simulink model "Mutant_19_of_purePursuitUSCityCopia"  (R2020a)
settings: Solver=FixedStepAuto  StartTime=0.0  StopTime=Ts  FixedStep=0.001  RelTol=1e-3
PreLoadFcn:
  | setUpPurePursuitUSCity
model workspace (MAT data in the model file):
  firstWarning = 0
  originalScenarioChecksum = 'F73A6DA3C723D3CA73A6F931B7A52A9C'
undefined symbols (not defined in the file): angVelGain, approximationReductionGain, L, ld, magnitude, minimalSpeed, nominalSpeed, psi_1, psi_2, psi_o, slope_x1, slope_x2, slope_y1, slope_y2, x_1, x_2, X_o, xRef, y_1, y_2, Y_o, yRef
libraries: simulink x15, autolibutils x4, autolibshared x3, robotalgslib x1
(part 3 of 3)

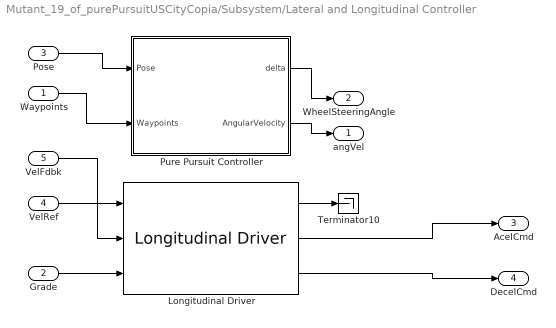
== system Mutant_19_of_purePursuitUSCityCopia/Subsystem/Lateral and Longitudinal Controller ==
  Waypoints : Inport
  Grade : Inport  Port=2
  Pose : Inport  Port=3
  VelRef : Inport  Port=4
  VelFdbk : Inport  Port=5
  Longitudinal Driver : autolibshared/Longitudinal Driver  extAccelOvr=off  extDecelOvr=off  extAccelHld=off  extDecelHld=off  extAccelZero=off  extDecelZero=off  cntrlType=PI  shftType=None  velUnits=m/s  gearOut=off  Kp=700  Ki=1  Kff=.1  Kg=0  VehVelVec=[0 100]  KffVec=[.1 .1]  KpVec=[10 10]  KiVec=[5 5]  KgVec=[0 0]  m=1500  Kpt=3000  tau=.1  L=2  aR=200  bR=2.5  cR=.5  g=9.81  vnom=9  Kaw=1  tauerr=.01  tauPt=2  GearInit=0  tShift=.1  pdlVec=[0.1 0.4 0.5 0.9]  upShftTbl=[-1 12.9375 26.4375 39.9375 51.18749999999999 62.4375 72.84375 83.25;-1 16.3125 29.8125 43.3125 54.5624 65.8125 76.78125 87.75;-1 19.6875 33.1875 46.68749999999999 57.9375 69.1875 80.71875 92.25;-1 33 52.5 77.25 100.5 138.75 161.875 185]  dwnShftTbl=[1 9.5625 23.0625 36.5625 47.8125 59.0625 68.90625 78.75;1 12.9375 26.4375 39.9375 51.18749999999999 62.4375 72.84375 83.25;1 16.3125 29.8125 43.3125 54.562499 65.8125 76.78125 87.75;1 19.6875 33.1875 46.68749999999999 57.9375 69.1875 80.71875 92.25]  tClutch=.5  tRev=.5  tPark=120  aMode=2  UpGearVec="[0  1  2  3  4  5  6  7]"  DownGearVec="[1  2  3  4  5  6  7  8]"
      settings: SourceProductBaseCode=PW,MT,VE,VP
  Pure Pursuit Controller : Subsystem
  Terminator10 : Terminator
  angVel : Outport
  WheelSteeringAngle : Outport  Port=2
  AcelCmd : Outport  Port=3
  DecelCmd : Outport  Port=4
  wires:
  Pure Pursuit Controller/1(delta) -> WheelSteeringAngle/1
  Waypoints/1 -> Pure Pursuit Controller/2(Waypoints)
  Pose/1 -> Pure Pursuit Controller/1(Pose)
  Grade/1 -> Longitudinal Driver/3
  VelRef/1 -> Longitudinal Driver/1
  VelFdbk/1 -> Longitudinal Driver/2
  Longitudinal Driver/1 -> Terminator10/1
  Pure Pursuit Controller/2(AngularVelocity) -> angVel/1
  Longitudinal Driver/2 -> AcelCmd/1
  Longitudinal Driver/3 -> DecelCmd/1

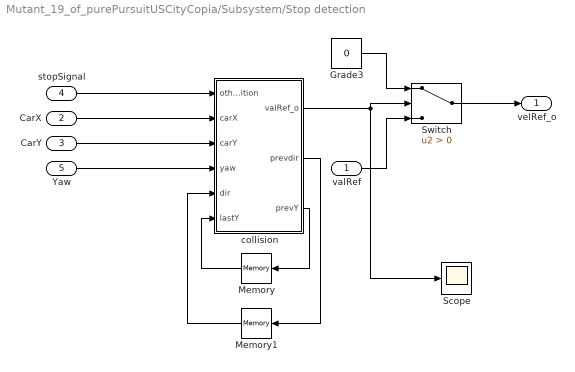
== system Mutant_19_of_purePursuitUSCityCopia/Subsystem/Stop detection ==
  valRef : Inport
  CarX : Inport  Port=2
  CarY : Inport  Port=3
  stopSignal : Inport  Port=4
  Yaw : Inport  Port=5
  Grade3 : Constant  Value=0
  Memory : Memory
  Memory1 : Memory
  Scope : Scope
  Switch : Switch  Criteria=u2 > Threshold
  collision : MATLAB Function  TreatAsAtomicUnit=on
  velRef_o : Outport
  wires:
  Switch/1 -> velRef_o/1
  valRef/1 -> Switch/3
  Grade3/1 -> Switch/1
  collision/1(valRef_o) -> Switch/2, Scope/1
  stopSignal/1 -> collision/1(otherCarPosition)
  CarX/1 -> collision/2(carX)
  CarY/1 -> collision/3(carY)
  Yaw/1 -> collision/4(yaw)
  collision/2(prevdir) -> Memory1/1
  collision/3(prevY) -> Memory/1
  Memory/1 -> collision/6(lastY)
  Memory1/1 -> collision/5(dir)

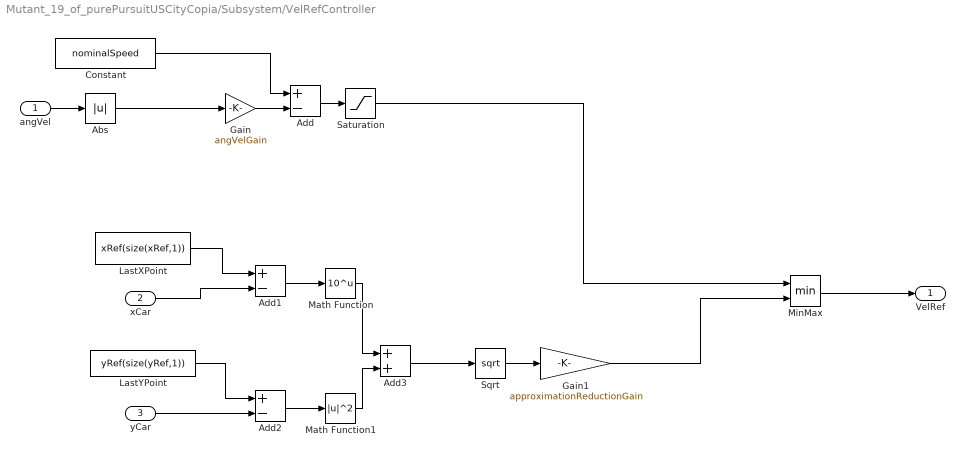
== system Mutant_19_of_purePursuitUSCityCopia/Subsystem/VelRefController ==
  angVel : Inport
  xCar : Inport  Port=2
  yCar : Inport  Port=3
  Abs : Abs
  Add : Sum  Inputs=+-
  Add1 : Sum  Inputs=+-
  Add2 : Sum  Inputs=+-
  Add3 : Sum
  Constant : Constant  Value=nominalSpeed
  Gain : Gain  Gain=angVelGain
  Gain1 : Gain  Gain=approximationReductionGain
  LastXPoint : Constant  Value=xRef(size(xRef,1))  SampleTime=0.1
  LastYPoint : Constant  Value=yRef(size(yRef,1))  SampleTime=0.1
  Math Function : Math  Operator=10^u  SaturateOnIntegerOverflow=on
  Math Function1 : Math  Operator=magnitude^2  SaturateOnIntegerOverflow=on
  MinMax : MinMax  Inputs=2
  Saturation : Saturate  UpperLimit=15  LowerLimit=minimalSpeed
  Sqrt : Sqrt  SaturateOnIntegerOverflow=on
  VelRef : Outport
  wires:
  angVel/1 -> Abs/1
  Gain/1 -> Add/2
  Abs/1 -> Gain/1
  Constant/1 -> Add/1
  Add/1 -> Saturation/1
  LastYPoint/1 -> Add2/1
  Math Function1/1 -> Add3/2
  Add3/1 -> Sqrt/1
  LastXPoint/1 -> Add1/1
  Math Function/1 -> Add3/1
  Add2/1 -> Math Function1/1
  yCar/1 -> Add2/2
  Add1/1 -> Math Function/1
  Sqrt/1 -> Gain1/1
  xCar/1 -> Add1/2
  Gain1/1 -> MinMax/2
  Saturation/1 -> MinMax/1
  MinMax/1 -> VelRef/1

== system Mutant_19_of_purePursuitUSCityCopia/Powertrain & Driveline/Driveline/AWD ==
  TPowertrain : Inport
  AWD : Gain  Gain=[1;1;1;1]./2
  TAxles : Outport  VectorParamsAs1DForOutWhenUnconnected=off
  wires:
  TPowertrain/1 -> AWD/1
  AWD/1 -> TAxles/1

== system Mutant_19_of_purePursuitUSCityCopia/Powertrain & Driveline/Driveline/FWD ==
  TPowertrain : Inport
  FWD : Gain  Gain=[1;1;0;0]
  TAxles : Outport  VectorParamsAs1DForOutWhenUnconnected=off
  wires:
  FWD/1 -> TAxles/1
  TPowertrain/1 -> FWD/1

== system Mutant_19_of_purePursuitUSCityCopia/Powertrain & Driveline/Driveline/RWD ==
  TPowertrain : Inport
  RWD : Gain  Gain=[0;0;1;1]
  TAxles : Outport  VectorParamsAs1DForOutWhenUnconnected=off
  wires:
  TPowertrain/1 -> RWD/1
  RWD/1 -> TAxles/1

== system Mutant_19_of_purePursuitUSCityCopia/Subsystem/Lateral and Longitudinal Controller/Pure Pursuit Controller ==
  note: The subsystem implements a Pure Pursuit controller. The "Pure Pursuit" block calculates the target direction and the "Wheel Steering Angle Formulation" block calculates the wheel steering angle.
  Pose : Inport
  Waypoints : Inport  Port=2
  Pure Pursuit : robotalgslib/Pure Pursuit  DesiredLinearVelocity=0.5  MaxAngularVelocity=1.0  LookaheadDistance=ld  TargetDirPort=on  SimulateUsing=Code generation
  Terminator6 : Terminator
  Terminator7 : Terminator
  Wheel Steering Angle Formulation : Subsystem  mask{L=L, ld=ld}
      mask prompts: L "Bicycle length"; ld "Lookahead distance"
      mask TypeOptions L: Bicycle length/Value
      mask TypeOptions ld: Lookahead distance/Value
      mask Display:
      | image("GeometryMask.png")
      | port_label('input', 1, 'alpha')
      | port_label('output', 1, 'delta')
  delta : Outport
  AngularVelocity : Outport  Port=2
  wires:
  Wheel Steering Angle Formulation/1(Al) -> delta/1
  Pure Pursuit/3 -> Wheel Steering Angle Formulation/1(alpha)
  Waypoints/1 -> Pure Pursuit/2
  Pure Pursuit/2 -> AngularVelocity/1, Terminator7/1
  Pose/1 -> Pure Pursuit/1
  Pure Pursuit/1 -> Terminator6/1

== system Mutant_19_of_purePursuitUSCityCopia/Subsystem/Lateral and Longitudinal Controller/Pure Pursuit Controller/Wheel Steering Angle Formulation ==
  alpha : Inport
  Bicycle length : Constant  Value=L
  Constant : Constant  Value=2
  Divide : Product  Inputs=*/
  Lookahead distance : Constant  Value=ld
  Product : Product
  Product1 : Product
  Sine Wave : Sin  TimeSource=Use external signal  SampleTime=0
  Trigonometric Function : Trigonometry  Operator=atan
  Al : Outport
  wires:
  Sine Wave/1 -> Product1/2
  Bicycle length/1 -> Product/2
  Constant/1 -> Product/1
  Product1/1 -> Divide/1
  Product/1 -> Product1/1
  Divide/1 -> Trigonometric Function/1
  Trigonometric Function/1 -> Al/1
  alpha/1 -> Sine Wave/1
  Lookahead distance/1 -> Divide/2

== matlab function Mutant_19_of_purePursuitUSCityCopia/Subsystem/Stop detection/collision ==
  data: valRef_o output; otherCarPosition input; carX input; carY input; yaw input; prevdir output; prevY output; dir input; lastY input
function [valRef_o,prevdir,prevY] = fcn(otherCarPosition,carX,carY ,yaw, dir, lastY)
%     ret=0;
%     for i=1:(size(waypoints,2)/2)
%         if waypoints(1,2*i-1)-data(1,1)<10 && waypoints(1,2*i)-data(1,2)<10 && waypoints(1,2*i-1)-data(1,1)>-10 && waypoints(1,2*i)-data(1,2)>-10 
%             ret=1;
%         end
%     end
    detectedCar=0;
    i=1;
    distanceX=0;
    distanceY=0;
    while i<=(size(otherCarPosition,2)/2) && detectedCar==0
        distanceX=carX-otherCarPosition(1,(i*2)-1);
        distanceY=carY-otherCarPosition(1,i*2);
        if yaw >= (pi*0)-0.1 && yaw <= (pi*0)+0.1 && otherCarPosition(1,(i*2)-1)>carX && abs(distanceX)<20
            detectedCar=i;
        elseif yaw >= (pi*1.5)-0.1 && yaw <= (pi*1.5)+0.1 && otherCarPosition(1,(i*2))<carY && abs(distanceY)<20
            detectedCar=i;
        elseif yaw >= (pi*1)-0.1 && yaw <= (pi*1)+0.1 && otherCarPosition(1,(i*2)-1)<carX && abs(distanceX)<20
            detectedCar=i;
        elseif yaw >= (pi*0.5)-0.1 && yaw <= (pi*0.5)+0.1 && otherCarPosition(1,(i*2))>carY && abs(distanceY)<20
            detectedCar=i;
        end
        i=i+1;
    end
    if detectedCar~=0
        if dir==0 && yaw >= (pi*0)-0.1 && yaw <= (pi*0)+0.1 && distanceY>0
            prevdir=1;
            lastY=distanceY;
        elseif dir==0 && yaw >= (pi*0)-0.1 && yaw <= (pi*0)+0.1 && distanceY<0
            prevdir=2;
            lastY=distanceY;
        elseif dir==0 && yaw >= (pi*1.5)-0.1 && yaw <= (pi*1.5)+0.1 && distanceX>0
            prevdir=1;
            lastY=distanceX;
        elseif dir==0 && yaw >= (pi*1.5)-0.1 && yaw <= (pi*1.5)+0.1 && distanceX<0
            prevdir=2;
            lastY=distanceX;
        elseif dir==0 && yaw >= (pi*1)-0.1 && yaw <= (pi*1)+0.1 && distanceY<0
            prevdir=1;
            lastY=distanceY;
        elseif dir==0 && yaw >= (pi*1)-0.1 && yaw <= (pi*1)+0.1 && distanceY>0
            prevdir=2;
            lastY=distanceY;
        elseif dir==0 && yaw >= (pi*0.5)-0.1 && yaw <= (pi*0.5)+0.1 && distanceX<0
            prevdir=1;
            lastY=distanceX;
        elseif dir==0 && yaw >= (pi*0.5)-0.1 && yaw <= (pi*0.5)+0.1 && distanceX>0
            prevdir=2;
            lastY=distanceX;
        else
            prevdir=dir;
        end
        dist=distanceX^2+distanceY^2;
        if dist<=22^2 && yaw >= (pi*0)-0.1 && yaw <= (pi*0)+0.1 && dir==1 && distanceY>-1 && distanceY<=lastY
            prevY=distanceY;
            valRef_o=1;
        elseif dist<=22^2 && yaw >= (pi*0)-0.1 && yaw <= (pi*0)+0.1 && dir==2 && distanceY<2 && distanceY>=lastY
            valRef_o=1;
            prevY=distanceY;
        elseif dist<=22^2 && yaw >= (pi*1.5)-0.1 && yaw <= (pi*1.5)+0.1 && dir==1 && distanceX>-1 && distanceX<=lastY
            prevY=distanceX;
            valRef_o=1;
        elseif dist<=22^2 && yaw >= (pi*1.5)-0.1 && yaw <= (pi*1.5)+0.1 && dir==2 && distanceX<2 && distanceX>=lastY
            valRef_o=1;
            prevY=distanceX;
        elseif dist<=22^2 && yaw >= (pi*1)-0.1 && yaw <= (pi*1)+0.1 && dir==1 && distanceY<2 && distanceY>=lastY
            prevY=distanceY;
            valRef_o=1;
        elseif dist<=22^2 && yaw >= (pi*1)-0.1 && yaw <= (pi*1)+0.1 && dir==2 && distanceY>-1 && distanceY<=lastY
            valRef_o=1;
            prevY=distanceY;
        elseif dist<=22^2 && yaw >= (pi*0.5)-0.1 && yaw <= (pi*0.5)+0.1 && dir==1 && distanceX<2 && distanceX>=lastY
            prevY=distanceX;
            valRef_o=1;
        elseif dist<=22^2 && yaw >= (pi*0.5)-0.1 && yaw <= (pi*0.5)+0.1 && dir==2 && distanceX>-1 && distanceX<=lastY
            valRef_o=1;
            prevY=distanceX;
        else
            valRef_o=0;
            prevY=lastY;
        end
    else
        valRef_o=0;
        prevdir=0;
        prevY=lastY;
    end
end

== matlab function Mutant_19_of_purePursuitUSCityCopia/Oracle/MATLAB Function ==
  data: x input; y output; y input; xref input; yref input
function y = fcn(x, y, xref, yref)
    
    minDist = inf;
    idx = 1;
    for i=1:size(xref,1)
       d = sqrt(abs(x-xref(i))^2+abs(y-yref(i))^2);
       if d<minDist
           minDist = d;
           idx = i;
       end
    end
    numberOfPoints = 1000;
    if idx < size(xref,1)
        xvals = linspace(xref(idx),xref(idx+1),numberOfPoints);
        yvals = linspace(yref(idx),yref(idx+1),numberOfPoints);

        for i=1:size(xvals,2)
           d = sqrt(abs(x-xvals(i))^2+abs(y-yvals(i))^2);
           if d<minDist
               minDist = d;

           end
        end
    end
    if idx>1
        xvals = linspace(xref(idx),xref(idx-1),numberOfPoints);
        yvals = linspace(yref(idx),yref(idx-1),numberOfPoints);
        for i=1:size(xvals,2)
           d = sqrt(abs(x-xvals(i))^2+abs(y-yvals(i))^2);
           if d<minDist
               minDist = d;

           end
        end
    end

y = minDist;

== matlab function Mutant_19_of_purePursuitUSCityCopia/Oracle/CalcVehiclesDIstance1 ==
  data: xCar input; yCar input; dist output; otherVehicles input
function dist = fcn(xCar,yCar,otherVehicles)
    
    dist=1000;
    j=1;
    while j<=(size(otherVehicles,2)/2)
        dist2Car=((xCar-otherVehicles(1,(2*j)-1))^2)+((yCar-otherVehicles(1,2*j))^2);
        if dist > dist2Car
            dist=dist2Car;
        end
        j=j+1;

    end
    dist=sqrt(dist);
end
